simulink model "s4_boost"  (R2019b)
settings: Solver=VariableStepAuto  StartTime=0.0  StopTime=15
libraries: powerlib x9, powerlib_meascontrol x1
settings Model: Creator=MAHMUD  LastModifiedBy=MAHMUD

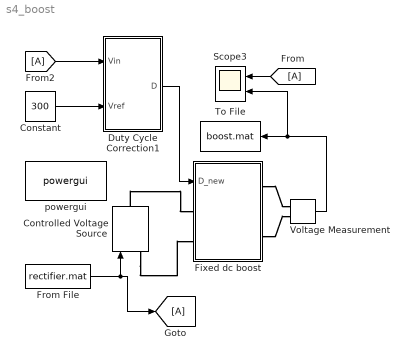
== system s4_boost ==
  Constant : Constant  Value=300
  Controlled Voltage Source : powerlib/Electrical Sources/Controlled Voltage Source  Initialize=on  Source_Type=DC  Amplitude=0  Phase=0  Frequency=0  Measurements=None
      settings: SourceProductName=Simscape Electrical
  Duty Cycle Correction1 : Subsystem
  Fixed dc boost : Subsystem
  From File : FromFile  FileName=rectifier.mat
  Scope3 : Scope  NumInputPorts=2
  To File : ToFile  Filename=boost.mat  SaveFormat=Timeseries
  Voltage Measurement : powerlib/Measurements/Voltage Measurement  PhasorSimulation=off  OutputType=Complex  PSBequivalent=0
      settings: SourceProductName=Simscape Electrical
  powergui : powerlib/powergui  Priority=1  SimulationMode=Continuous  SampleTime=1e-6  frequency=60  Iterations=50  frequencyindice=0  Pbase=100e6  ErrMax=1e-4  UnitsV=kV  UnitsW=MW  buscounter=0  FunctionMessages=off  echomessages=off  EnableUseOfTLC=off  CurrentSourceSwitches=off  DisableSnubberDevices=off  DisableRonSwitches=off  DisableVfSwitches=off  DisplayEquations=off  AutomaticDiscreteSolvers=off  SolverType=Tustin/Backward Euler (TBE)  Interpol=off  ExternalGateDelay=off  methode=off  Ts=100  x0status=blocks  SPID=on  SwTol=0  HookPort=off  NonlinearTolerance=1e-4  nMaxIteration=100  ContinueOnMaxIteration=off  RestoreLinks=warning  ResistiveCurrentMeasurement=off  Frange=[0:2:500]  Ylog=off  Xlog=on  ShowGrid=off  save=off  variable=ZData  structure=0  ZoomFFT=off  StartTime=0.0  cycles=1  DisplayStyle=1  fundamental=60  FreqAxis=off  MaxFrequency=1000  frequencyindicesteady=1  RmsSteady=1  display=off
      settings: SourceProductName=Simscape Electrical
  wires:
  Voltage Measurement/1 -> Scope3/2, To File/1
  [A] -> Duty Cycle Correction1/1(Vin)
  From File/1 -> [A], Controlled Voltage Source/1
  Duty Cycle Correction1/1(D) -> Fixed dc boost/1(D_new)
  Constant/1 -> Duty Cycle Correction1/2(Vref)
  [A] -> Scope3/1
  connections:
  Fixed dc boost/RConn2 -- Voltage Measurement/LConn2
  Fixed dc boost/RConn1 -- Voltage Measurement/LConn1
  Controlled Voltage Source/LConn1 -- Fixed dc boost/LConn2
  Controlled Voltage Source/RConn1 -- Fixed dc boost/LConn1

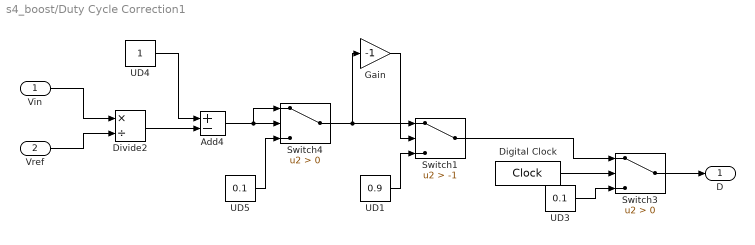
== system s4_boost/Duty Cycle Correction1 ==
  Vin : Inport
  Vref : Inport  Port=2
  Add4 : Sum  Inputs=+-
  Digital Clock : DigitalClock
  Divide2 : Product  Inputs=*/
  Gain : Gain  Gain=-1
  Switch1 : Switch  Criteria=u2 > Threshold  Threshold=-1  ZeroCross=off
  Switch3 : Switch  Criteria=u2 > Threshold  ZeroCross=off
  Switch4 : Switch  Criteria=u2 > Threshold  ZeroCross=off
  UD1 : Constant  Value=0.9
  UD3 : Constant  Value=0.1
  UD4 : Constant
  UD5 : Constant  Value=0.1
  D : Outport
  wires:
  Digital Clock/1 -> Switch3/2
  UD3/1 -> Switch3/3
  Vref/1 -> Divide2/2
  Divide2/1 -> Add4/2
  UD4/1 -> Add4/1
  Add4/1 -> Switch4/1, Switch4/2
  UD5/1 -> Switch4/3
  Vin/1 -> Divide2/1
  Switch3/1 -> D/1
  UD1/1 -> Switch1/3
  Switch4/1 -> Gain/1, Switch1/1
  Switch1/1 -> Switch3/1
  Gain/1 -> Switch1/2

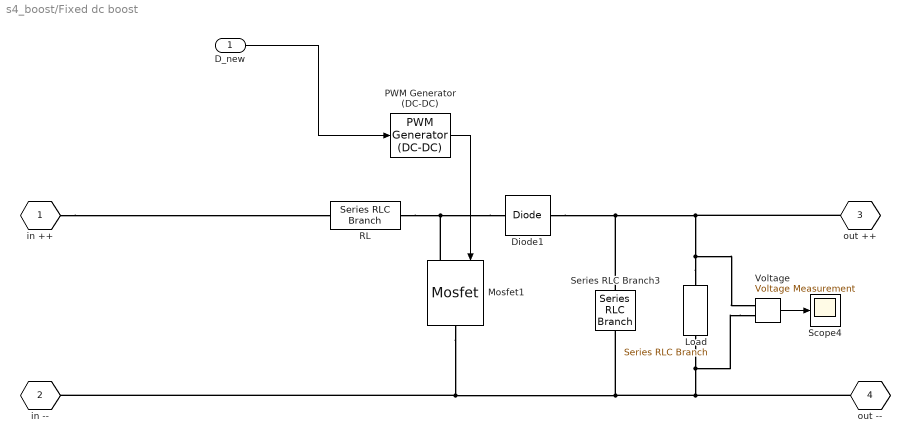
== system s4_boost/Fixed dc boost ==
  D_new : Inport
  Diode1 : powerlib/Power Electronics/Diode  Ron=1e-3  Lon=0  Vf=0  IC=0  UseSnubber=off  Rs=inf  Cs=inf  Measurements=off
      settings: SourceProductName=Simscape Electrical
  Load : powerlib/Elements/Series RLC Branch  LConnTagsString=__new0  RConnTagsString=__new0  BranchType=R  Resistance=3  Inductance=200e-6  SetiL0=off  InitialCurrent=0  Capacitance=400e-6  Setx0=off  InitialVoltage=0  Measurements=None
      settings: SourceProductName=Simscape Electrical
  Mosfet1 : powerlib/Power Electronics/Mosfet  Ron=1e-3  Lon=0  Rd=1e-3  Vfd=0  IC=0  Rs=inf  Cs=inf  Measurements=off
      settings: SourceProductName=Simscape Electrical
  PWM Generator (DC-DC) : powerlib_meascontrol/Pulse & Signal Generators/PWM Generator (DC-DC)  Fsw=1e3  Ts=0
      settings: SourceProductName=Simscape Electrical
  RL : powerlib/Elements/Series RLC Branch  LConnTagsString=__new0  RConnTagsString=__new0  BranchType=RL  Resistance=1e-3  Inductance=250e-6  SetiL0=off  InitialCurrent=0  Capacitance=1e-6  Setx0=off  InitialVoltage=0  Measurements=None
      settings: SourceProductName=Simscape Electrical
  Scope4 : Scope
  Series RLC Branch3 : powerlib/Elements/Series RLC Branch  LConnTagsString=__new0  RConnTagsString=__new0  BranchType=C  Resistance=1e-4  Inductance=200e-6  SetiL0=off  InitialCurrent=0  Capacitance=200e-3  Setx0=off  InitialVoltage=40  Measurements=None
      settings: SourceProductName=Simscape Electrical
  "Voltage " : powerlib/Measurements/Voltage Measurement  PhasorSimulation=off  OutputType=Complex  PSBequivalent=0
      settings: SourceProductName=Simscape Electrical
  in ++ : PMIOPort  Tag=PMCPort  Side=Left
  in -- : PMIOPort  Tag=PMCPort  Port=2  Side=Left
  out ++ : PMIOPort  Tag=PMCPort  Port=3  Side=Right
  out -- : PMIOPort  Tag=PMCPort  Port=4  Side=Right
  wires:
  "Voltage "/1 -> Scope4/1
  PWM Generator (DC-DC)/1 -> Mosfet1/1
  D_new/1 -> PWM Generator (DC-DC)/1
  connections:
  Load/LConn1 -- Series RLC Branch3/LConn1 -- Diode1/RConn1 -- out ++/RConn1 -- "Voltage "/LConn1
  "Voltage "/LConn2 -- Load/RConn1 -- out --/RConn1 -- Mosfet1/RConn1 -- in --/RConn1 -- Series RLC Branch3/RConn1
  Diode1/LConn1 -- RL/RConn1 -- Mosfet1/LConn1
  in ++/RConn1 -- RL/LConn1
